simulink model "sampleModel1858_1_sub_sub"  (R2023a)
settings: Solver=VariableStepAuto  StartTime=0.0  StopTime=10.0  RelTol=1e-3
libraries: hdlsllib x5, simulink x1
settings Model: Creator=user1  LastModifiedBy=user1

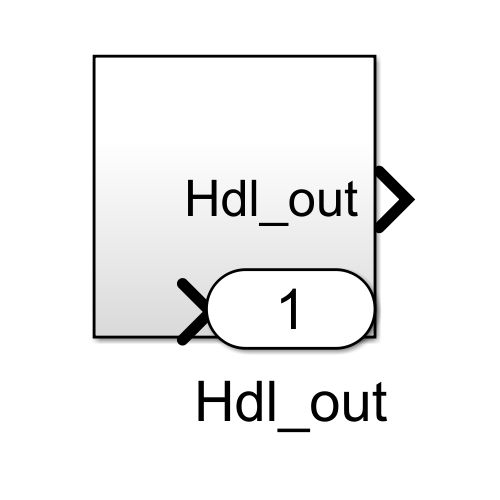
[thumbnail: Simulink's stored preview of the top-level diagram]
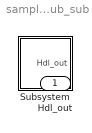
== system sampleModel1858_1_sub_sub ==
  Subsystem : Subsystem
  Hdl_out : Outport  OutDataTypeStr=uint8

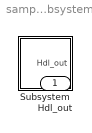
== system sampleModel1858_1_sub_sub/Subsystem ==
  Subsystem : Subsystem
  Hdl_out : Outport  OutDataTypeStr=uint8

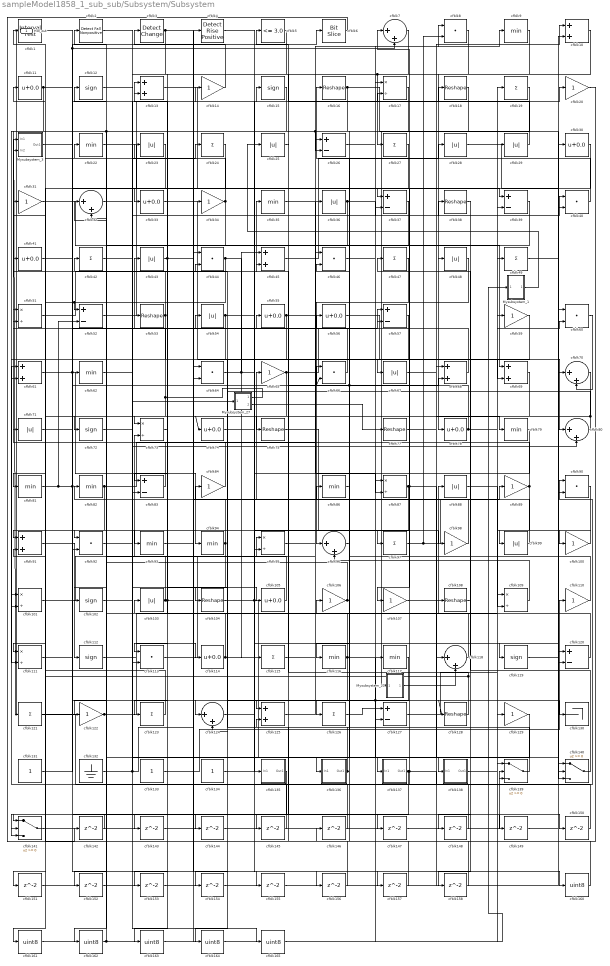
== system sampleModel1858_1_sub_sub/Subsystem/Subsystem ==
  Mysubsystem_1 : Subsystem  TreatAsAtomicUnit=on  RTWFcnName=Mysubsystem_1
      settings: RTWFcnNameOpts=User specified  RTWFileNameOpts=Use function name
  Mysubsystem_20 : Subsystem  TreatAsAtomicUnit=on  RTWFcnName=Mysubsystem_20
      settings: RTWFcnNameOpts=User specified  RTWFileNameOpts=Use function name
  Mysubsystem_27 : Subsystem  TreatAsAtomicUnit=on  RTWFcnName=Mysubsystem_27
      settings: RTWFcnNameOpts=User specified  RTWFileNameOpts=Use function name
  Mysubsystem_3 : Subsystem  TreatAsAtomicUnit=on  RTWFcnName=Mysubsystem_3
      settings: RTWFcnNameOpts=User specified  RTWFileNameOpts=Use function name
  cfblk1 : hdlsllib/Logic and Bit Operations/Interval Test  IntervalClosedRight=on  uplimit=0.5  IntervalClosedLeft=on  lowlimit=-0.5  OutDataTypeStr=uint8
  cfblk{10,13,45,61,68..69,91,125} (8 alike) : Sum  OutDataTypeStr=uint8
  cfblk{14,20,31,34,59,65,84,89,98,100,106..107,110,122,129} (15 alike) : Gain  OutDataTypeStr=uint8
  cfblk{17,51,73,87,95,101,109,111} (8 alike) : Product  Inputs=*/  OutDataTypeStr=uint8  RndMeth=Zero  SaturateOnIntegerOverflow=on
  cfblk{12,15,72,102,112,119} (6 alike) : Signum
  cfblk{23,25,28..29,36,43,48,54,67,71,88,99,103} (13 alike) : Abs  OutDataTypeStr=uint8  SaturateOnIntegerOverflow=off
  cfblk{16,18,38,53,75,77,104,108,128} (9 alike) : Reshape
  cfblk{11,30,33,41,55..56,74,78,105,114} (10 alike) : Bias  Bias=0.0  SaturateOnIntegerOverflow=off
  cfblk{8,40,44,46,60,64,66,90,92,113} (10 alike) : DotProduct  OutDataTypeStr=uint8
  cfblk{19,24,27,42,47,49,97,115,121,123,126} (11 alike) : Sum  Inputs=+  OutDataTypeStr=uint8
  cfblk{9,22,35,62,79,81..82,86,93..94,116..117} (12 alike) : MinMax  OutDataTypeStr=uint8
  cfblk{7,32,70,80,96,118,124} (7 alike) : Sum  Inputs=|++  OutDataTypeStr=uint8
  cfblk{26,37,39,52,57,83,120,127} (8 alike) : Sum  Inputs=+-  OutDataTypeStr=uint8
  cfblk130 : Terminator
  cfblk131 : Constant  OutDataTypeStr=uint8  SampleTime=-1
  cfblk132 : Ground
  cfblk133 : Constant  OutDataTypeStr=uint8  SampleTime=-1
  cfblk134 : Constant  OutDataTypeStr=uint8  SampleTime=-1
  cfblk135 : Subsystem
      settings: LibrarySourceBlock=|
      | hdlsllib/Ports &
      | Subsystems/Subsystem
  cfblk136 : Subsystem
      settings: LibrarySourceBlock=|
      | hdlsllib/Ports &
      | Subsystems/Subsystem
  cfblk137 : Subsystem
      settings: LibrarySourceBlock=|
      | hdlsllib/Ports &
      | Subsystems/Subsystem
  cfblk138 : Subsystem
      settings: LibrarySourceBlock=|
      | hdlsllib/Ports &
      | Subsystems/Subsystem
  cfblk139 : Switch  OutDataTypeStr=uint8  SaturateOnIntegerOverflow=off  InputSameDT=off
  cfblk140 : Switch  OutDataTypeStr=uint8  SaturateOnIntegerOverflow=off  InputSameDT=off
  cfblk141 : Switch  OutDataTypeStr=uint8  SaturateOnIntegerOverflow=off  InputSameDT=off
  cfblk{142..158} (17 alike) : Delay  SampleTime=1
  cfblk{160..165} (6 alike) : DataTypeConversion  OutDataTypeStr=uint8  SaturateOnIntegerOverflow=off  RndMeth=Floor
  cfblk2 : hdlsllib/Logic and Bit Operations/Detect Fall Nonpositive  vinit=0  OutDataTypeStr=uint8
  cfblk3 : simulink/Logic and Bit Operations/Detect Change  vinit=0  OutDataTypeStr=uint8
      settings: LibrarySourceBlock=|
      | hdlsllib/Logic and Bit
      | Operations/Detect
      | Change
  cfblk4 : hdlsllib/Logic and Bit Operations/Detect Rise Positive  vinit=0  OutDataTypeStr=uint8
  cfblk5 : hdlsllib/Logic and Bit Operations/Compare To Constant  relop=<=  const=3.0  OutDataTypeStr=uint8
  cfblk6 : hdlsllib/Logic and Bit Operations/Bit Slice  lidx=7  ridx=0
  Hdl_out : Outport  OutDataTypeStr=uint8
  wires:
  Mysubsystem_27/2(Out2) -> cfblk77/1
  Mysubsystem_27/1(Out1) -> cfblk1/1, cfblk73/1
  Mysubsystem_20/1(Out1) -> cfblk118/2
  cfblk18/1 -> Mysubsystem_20/1(In1)
  Mysubsystem_3/1(Out1) -> cfblk144/1
  Mysubsystem_1/1(Out1) -> cfblk25/1
  cfblk164/1 -> Mysubsystem_1/1(In1)
  cfblk165/1 -> cfblk117/1
  cfblk2/1 -> cfblk165/1
  cfblk117/1 -> cfblk164/1
  cfblk163/1 -> cfblk129/1
  cfblk5/1 -> cfblk163/1
  cfblk162/1 -> cfblk44/1, cfblk82/1
  cfblk161/1 -> cfblk4/1
  cfblk24/1 -> cfblk161/1
  cfblk160/1 -> cfblk66/2, cfblk56/1
  cfblk158/1 -> cfblk125/2
  cfblk38/1 -> cfblk158/1
  cfblk157/1 -> cfblk46/2
  cfblk156/1 -> cfblk51/2
  cfblk71/1 -> cfblk156/1
  cfblk155/1 -> cfblk68/1
  cfblk12/1 -> cfblk155/1
  cfblk154/1 -> cfblk90/2
  cfblk153/1 -> cfblk87/1
  cfblk27/1 -> cfblk153/1
  cfblk152/1 -> cfblk64/1
  cfblk151/1 -> cfblk37/2
  cfblk150/1 -> cfblk101/1
  cfblk74/1 -> cfblk150/1
  cfblk149/1 -> cfblk10/2
  cfblk124/1 -> cfblk149/1
  cfblk148/1 -> cfblk7/1
  cfblk108/1 -> cfblk148/1
  cfblk147/1 -> cfblk39/2
  cfblk146/1 -> cfblk32/1
  cfblk20/1 -> cfblk146/1
  cfblk145/1 -> cfblk61/1
  cfblk25/1 -> cfblk145/1
  cfblk144/1 -> cfblk127/2
  cfblk143/1 -> cfblk139/1
  cfblk73/1 -> cfblk143/1
  cfblk142/1 -> cfblk141/1
  cfblk6/1 -> cfblk142/1
  cfblk29/1 -> cfblk5/1
  cfblk82/1 -> cfblk46/1, cfblk91/1
  cfblk59/1 -> cfblk104/1
  cfblk42/1 -> cfblk14/1
  cfblk109/1 -> cfblk96/2
  cfblk137/1(Out1) -> cfblk139/3, cfblk17/2, cfblk141/3
  cfblk39/1 -> cfblk126/1
  cfblk55/1 -> cfblk69/2, cfblk83/1
  cfblk10/1 -> cfblk125/1
  cfblk79/1 -> cfblk95/2
  cfblk60/1 -> cfblk70/2
  cfblk35/1 -> cfblk87/2
  cfblk70/1 -> cfblk81/1
  cfblk54/1 -> cfblk70/1, cfblk92/2
  cfblk51/1 -> cfblk35/1
  cfblk107/1 -> cfblk140/2
  cfblk135/1(Out1) -> cfblk141/2
  cfblk64/1 -> cfblk98/1, cfblk45/1
  cfblk57/1 -> cfblk101/2
  cfblk43/1 -> cfblk123/1, cfblk157/1
  cfblk141/1 -> cfblk139/2
  cfblk26/1 -> cfblk9/1
  cfblk37/1 -> cfblk102/1
  cfblk90/1 -> cfblk100/1
  cfblk36/1 -> cfblk64/2, cfblk40/2
  cfblk92/1 -> cfblk40/1
  cfblk106/1 -> cfblk66/1, cfblk22/1
  cfblk114/1 -> cfblk13/1, cfblk18/1
  cfblk115/1 -> cfblk119/1
  cfblk101/1 -> cfblk95/1
  cfblk116/1 -> cfblk128/1, cfblk140/3, cfblk54/1, cfblk124/2
  cfblk30/1 -> cfblk107/1
  cfblk19/1 -> cfblk136/1(In1)
  cfblk41/1 -> cfblk6/1, cfblk7/2
  cfblk62/1 -> cfblk80/2
  cfblk88/1 -> cfblk109/1
  cfblk139/1 -> cfblk41/1
  cfblk112/1 -> cfblk114/1
  cfblk72/1 -> cfblk105/1
  cfblk96/1 -> cfblk26/1
  cfblk65/1 -> cfblk17/1, cfblk154/1
  cfblk127/1 -> cfblk29/1
  cfblk32/1 -> cfblk138/1(In1)
  cfblk134/1 -> cfblk106/1
  cfblk40/1 -> cfblk16/1
  cfblk102/1 -> cfblk24/1
  cfblk44/1 -> cfblk52/1, cfblk151/1, cfblk115/1
  cfblk69/1 -> cfblk122/1
  cfblk84/1 -> cfblk31/1
  cfblk34/1 -> cfblk11/1, cfblk92/1
  cfblk125/1 -> cfblk36/1
  cfblk118/1 -> cfblk32/2
  cfblk11/1 -> cfblk130/1, cfblk111/2
  cfblk28/1 -> cfblk140/1
  cfblk138/1(Out1) -> cfblk19/1
  cfblk14/1 -> cfblk3/1
  cfblk123/1 -> cfblk71/1
  cfblk17/1 -> cfblk26/2, cfblk152/1
  cfblk48/1 -> cfblk97/1
  cfblk16/1 -> cfblk93/1, cfblk120/1
  cfblk93/1 -> cfblk38/1
  cfblk122/1 -> cfblk49/1, Hdl_out/1
  cfblk45/1 -> cfblk28/1
  cfblk13/1 -> cfblk37/1
  cfblk75/1 -> cfblk118/1
  cfblk83/1 -> cfblk51/1
  cfblk105/1 -> cfblk12/1
  cfblk131/1 -> cfblk62/1
  cfblk56/1 -> cfblk80/1
  cfblk9/1 -> cfblk27/1, cfblk113/2
  cfblk3/1 -> cfblk83/2, cfblk147/1
  cfblk33/1 -> cfblk67/1
  cfblk111/1 -> cfblk57/1
  cfblk100/1 -> cfblk99/1
  cfblk4/1 -> cfblk160/1
  cfblk87/1 -> cfblk108/1, cfblk57/2, cfblk111/1
  cfblk113/1 -> cfblk20/1
  cfblk104/1 -> cfblk137/1(In1), cfblk120/2
  cfblk95/1 -> cfblk8/1
  cfblk78/1 -> cfblk60/2, cfblk45/2
  cfblk132/1 -> Mysubsystem_27/1(In1), cfblk34/1
  cfblk128/1 -> cfblk55/1, cfblk91/2
  cfblk1/1 -> cfblk39/1
  cfblk81/1 -> cfblk124/1, cfblk13/2, cfblk52/2
  cfblk94/1 -> cfblk2/1, cfblk113/1
  cfblk46/1 -> cfblk48/1
  cfblk80/1 -> cfblk74/1, cfblk44/2
  cfblk66/1 -> cfblk43/1
  cfblk136/1(Out1) -> cfblk103/1, cfblk86/1
  cfblk91/1 -> cfblk112/1
  cfblk98/1 -> cfblk42/1
  cfblk97/1 -> cfblk59/1, cfblk8/2
  cfblk7/1 -> cfblk75/1
  cfblk68/1 -> cfblk23/1
  cfblk119/1 -> cfblk30/1
  cfblk89/1 -> Mysubsystem_3/2(In2), cfblk109/2
  cfblk103/1 -> cfblk53/1, cfblk89/1, cfblk73/2
  cfblk22/1 -> cfblk135/1(In1)
  cfblk23/1 -> cfblk33/1
  cfblk49/1 -> cfblk60/1
  cfblk121/1 -> cfblk90/1
  cfblk86/1 -> cfblk116/1
  cfblk53/1 -> Mysubsystem_3/1(In1), cfblk61/2
  cfblk133/1 -> cfblk110/1
  cfblk110/1 -> cfblk84/1
  cfblk126/1 -> cfblk127/1
  cfblk99/1 -> cfblk65/1
  cfblk140/1 -> cfblk47/1
  cfblk61/1 -> cfblk94/1, cfblk68/2
  cfblk129/1 -> cfblk162/1
  cfblk67/1 -> cfblk10/1
  cfblk52/1 -> cfblk15/1
  cfblk120/1 -> cfblk88/1
  cfblk15/1 -> cfblk121/1, cfblk72/1
  cfblk77/1 -> cfblk79/1
  cfblk8/1 -> cfblk78/1
  cfblk31/1 -> cfblk69/1
  cfblk47/1 -> cfblk96/1

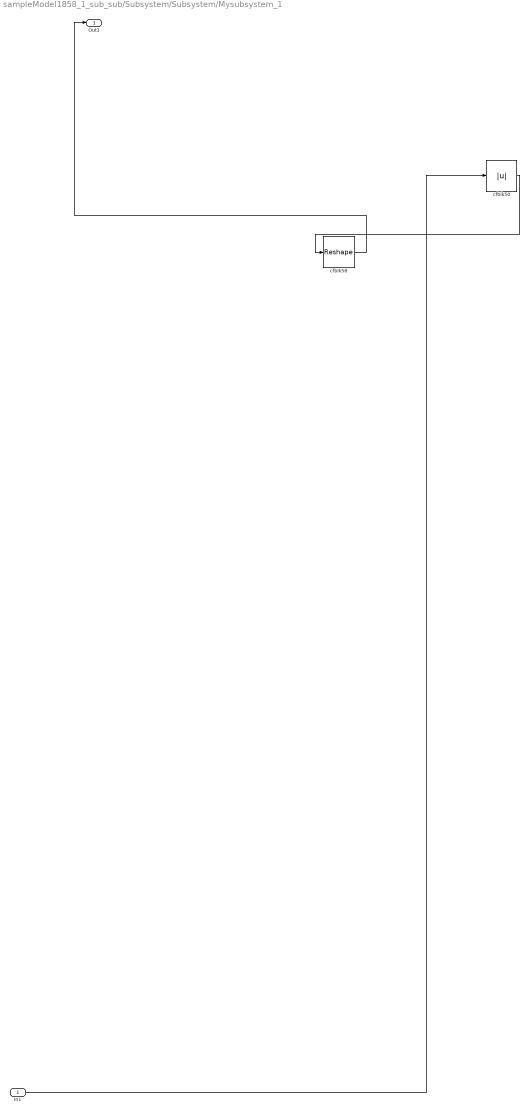
== system sampleModel1858_1_sub_sub/Subsystem/Subsystem/Mysubsystem_1 ==
  In1 : Inport
  cfblk50 : Abs  SaturateOnIntegerOverflow=off
  cfblk58 : Reshape
  Out1 : Outport
  wires:
  cfblk50/1 -> cfblk58/1
  cfblk58/1 -> Out1/1
  In1/1 -> cfblk50/1

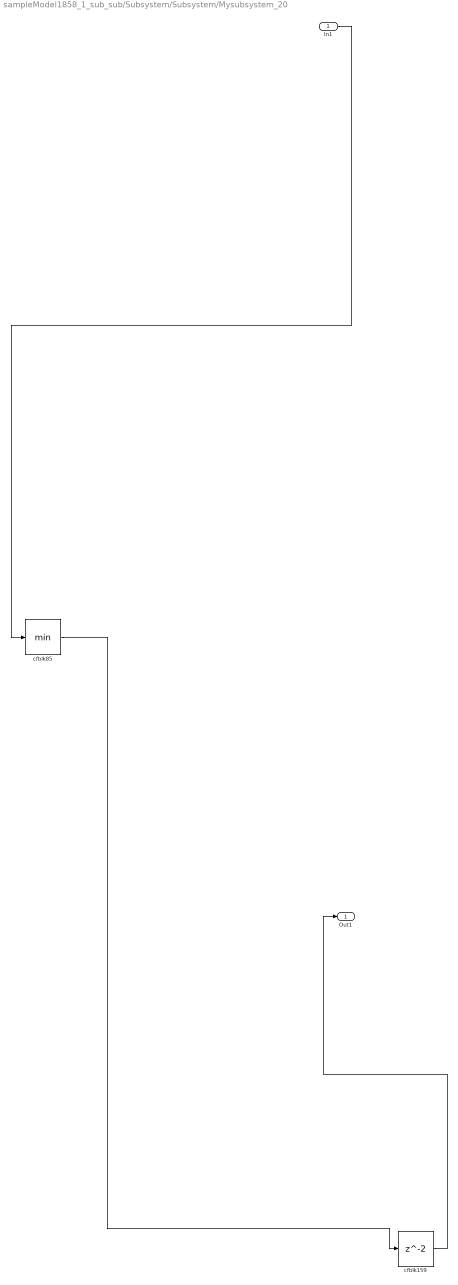
== system sampleModel1858_1_sub_sub/Subsystem/Subsystem/Mysubsystem_20 ==
  In1 : Inport
  cfblk159 : Delay  SampleTime=1
  cfblk85 : MinMax
  Out1 : Outport
  wires:
  cfblk85/1 -> cfblk159/1
  cfblk159/1 -> Out1/1
  In1/1 -> cfblk85/1

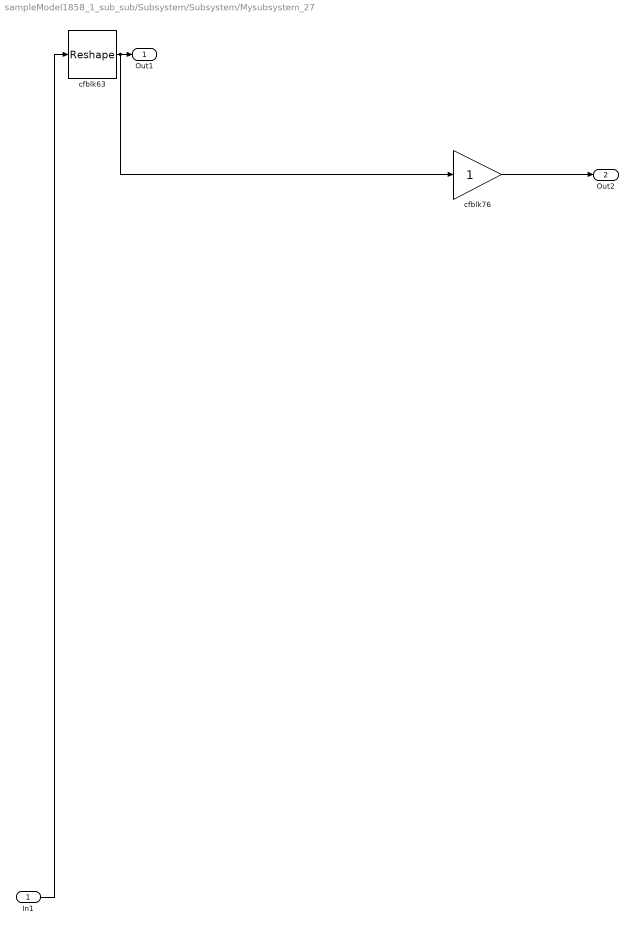
== system sampleModel1858_1_sub_sub/Subsystem/Subsystem/Mysubsystem_27 ==
  In1 : Inport
  cfblk63 : Reshape
  cfblk76 : Gain
  Out1 : Outport
  Out2 : Outport  Port=2
  wires:
  In1/1 -> cfblk63/1
  cfblk63/1 -> cfblk76/1, Out1/1
  cfblk76/1 -> Out2/1

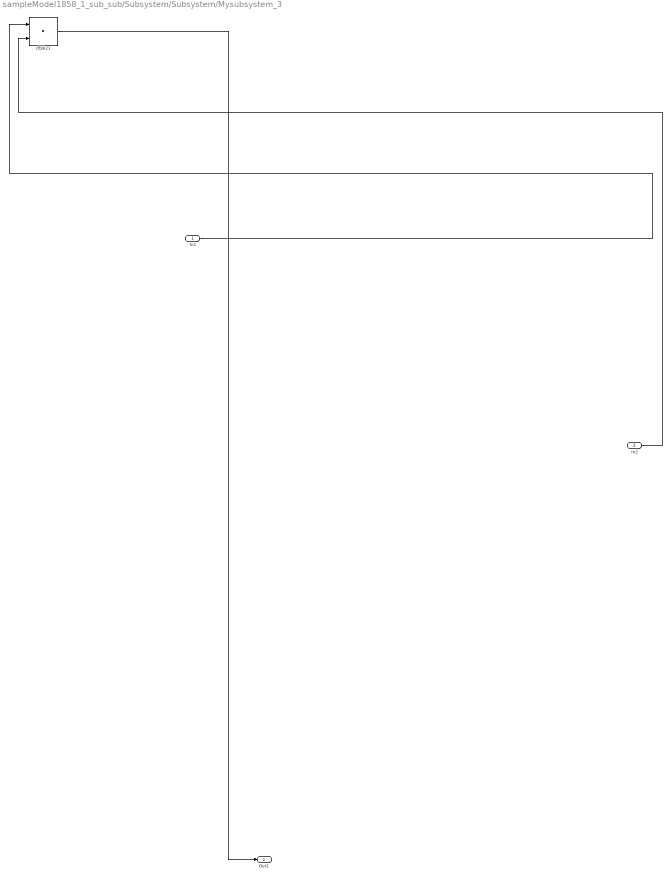
== system sampleModel1858_1_sub_sub/Subsystem/Subsystem/Mysubsystem_3 ==
  In1 : Inport
  In2 : Inport  Port=2
  cfblk21 : DotProduct  OutDataTypeStr=Inherit: Inherit via internal rule
  Out1 : Outport
  wires:
  In1/1 -> cfblk21/1
  cfblk21/1 -> Out1/1
  In2/1 -> cfblk21/2

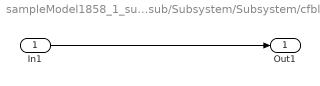
== system sampleModel1858_1_sub_sub/Subsystem/Subsystem/cfblk135 ==
  In1 : Inport
  Out1 : Outport
  wires:
  In1/1 -> Out1/1

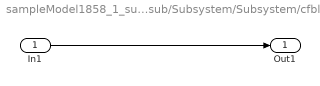
== system sampleModel1858_1_sub_sub/Subsystem/Subsystem/cfblk136 ==
  In1 : Inport
  Out1 : Outport
  wires:
  In1/1 -> Out1/1

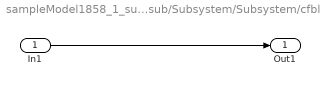
== system sampleModel1858_1_sub_sub/Subsystem/Subsystem/cfblk137 ==
  In1 : Inport
  Out1 : Outport
  wires:
  In1/1 -> Out1/1

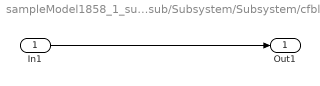
== system sampleModel1858_1_sub_sub/Subsystem/Subsystem/cfblk138 ==
  In1 : Inport
  Out1 : Outport
  wires:
  In1/1 -> Out1/1
